simulink model "Punto_7"  (R2023a)
settings: Solver=VariableStepAuto  StartTime=0.0  StopTime=50  RelTol=1e-3
settings Model: Creator=laura  LastModifiedBy=laura

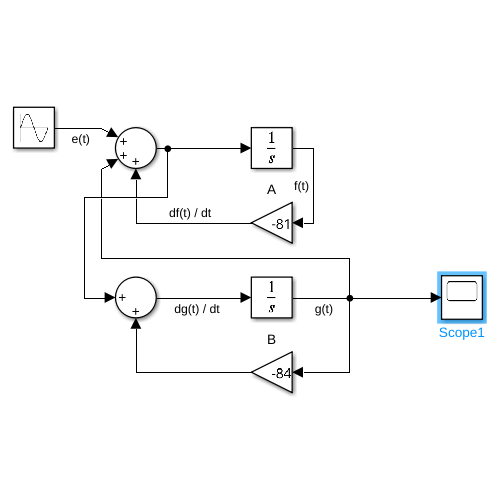
[thumbnail: Simulink's stored preview of the top-level diagram]
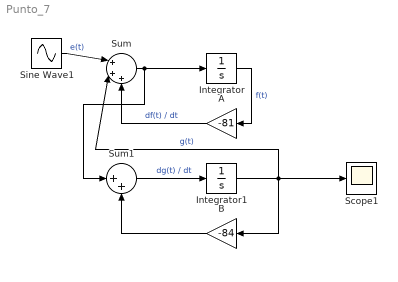
== system Punto_7 ==
  A : Gain  Gain=-81
  B : Gain  Gain=-84
  Integrator : Integrator
  Integrator1 : Integrator
  Scope1 : Scope
  Sine Wave1 : Sin  Frequency=[84 3*84 9*84 15*84 200*84 1000*84]  Phase=81/2*pi*[84 3*84 9*84 15*84 200*84 1000*84]  SampleTime=0
  Sum : Sum  Inputs=|+++
  Sum1 : Sum  Inputs=|++
  wires:
  Integrator/1 -> A/1  "f(t)"
  Integrator1/1 -> Sum/2, Scope1/1, B/1  "g(t)"
  Sum1/1 -> Integrator1/1  "dg(t) / dt"
  A/1 -> Sum/3  "df(t) / dt"
  B/1 -> Sum1/2
  Sum/1 -> Integrator/1, Sum1/1
  Sine Wave1/1 -> Sum/1  "e(t)"
